simulink model "TrafficLights"  (R2023b)
settings: Solver=FixedStepAuto  StartTime=0.0  StopTime=50  FixedStep=1e-3  RelTol=1e-3  EnableMultiTasking=on
libraries: arduinolib x4
settings Model: ExtModeTrigDuration=2  Creator=MOHAMED  LastModifiedBy=MOHAMED
settings OptimizationCC: EnhancedBackFolding=on  PassReuseOutputArgsAs=Individual arguments  ZeroExternalMemoryAtStartup=off  ZeroInternalMemoryAtStartup=off  MaxStackSize=64  OptimizeBlockOrder=speed  DifferentSizesBufferReuse=on  OptimizationCustomize=off  EfficientTunableParamExpr=on
settings DebuggingCC: ParameterTunabilityLossMsg=error
settings HardwareCC: ProdBitPerInt=16  ProdBitPerPointer=16  ProdBitPerSizeT=16  ProdBitPerPtrDiffT=16  ProdLargestAtomicFloat=None  ProdWordSize=8  ProdHWDeviceType=Atmel->AVR
settings SFSimCC: MATLABDynamicMemAlloc=off
settings RTWCC: Description=Embedded Coder  SystemTargetFile=ert.tlc  HardwareBoard=Arduino Uno  TemplateMakefile=ert_default_tmf  Toolchain=Arduino AVR  BuildConfiguration=Faster Runs
settings CodeAppCC: ForceParamTrailComments=on  IgnoreCustomStorageClasses=off  OperatorAnnotations=on  SimulinkDataObjDesc=on  SFDataObjDesc=on  InsertBlockDesc=on
settings ERTTargetCC: SupportContinuousTime=on  SupportVariableSizeSignals=on  ExtModeTransport=3  ExtModeStaticAlloc=on  ExtModeAutomaticAllocSize=off  ExtModeStaticAllocSize=250  ExtModeMexFile=ext_xcp  ExtModeIntrfLevel=Level2 - Open

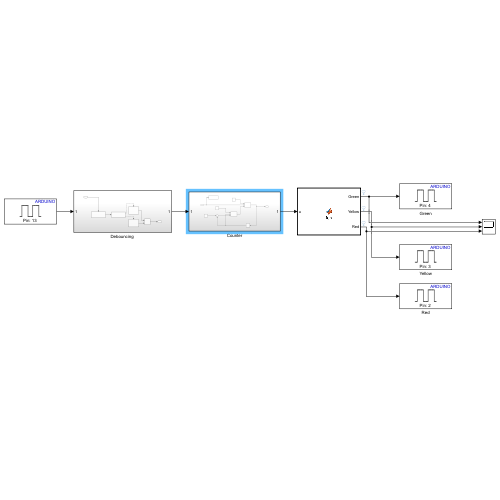
[thumbnail: Simulink's stored preview of the top-level diagram]
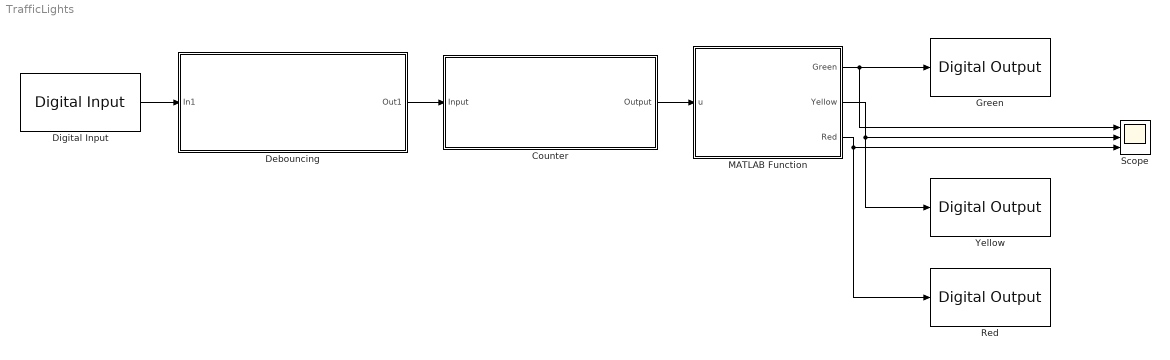
== system TrafficLights ==
  Counter : Subsystem
  "Debouncing " : Subsystem
  Digital Input : arduinolib/Digital Input  pinNumber=13  mode=Default  Direction=input  SampleTime=0.1  blockPlatform=arduino
  Green : arduinolib/Digital Output  pinNumber=4  Direction=output  blockPlatform=arduino
  MATLAB Function : MATLAB Function  TreatAsAtomicUnit=on
  Red : arduinolib/Digital Output  pinNumber=2  Direction=output  blockPlatform=arduino
  Scope : Scope  NumInputPorts=3
  Yellow : arduinolib/Digital Output  pinNumber=3  Direction=output  blockPlatform=arduino
  wires:
  Digital Input/1 -> "Debouncing "/1(In1)
  MATLAB Function/1(Green) -> Scope/1, Green/1
  "Debouncing "/1(Out1) -> Counter/1(Input)
  Counter/1(Output) -> MATLAB Function/1(u)
  MATLAB Function/3(Red) -> Red/1, Scope/3
  MATLAB Function/2(Yellow) -> Yellow/1, Scope/2

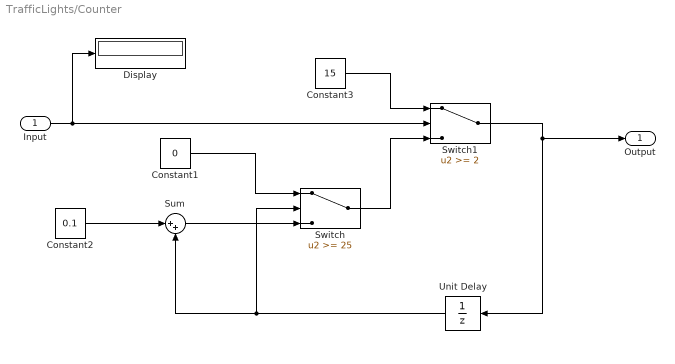
== system TrafficLights/Counter ==
  Input : Inport
  Constant1 : Constant  Value=0
  Constant2 : Constant  Value=0.1
  Constant3 : Constant  Value=15
  Display : Display
  Sum : Sum  Inputs=|++
  Switch : Switch  Threshold=25  SaturateOnIntegerOverflow=off  InputSameDT=off
  Switch1 : Switch  Threshold=2  SaturateOnIntegerOverflow=off  InputSameDT=off
  Unit Delay : UnitDelay  SampleTime=-1  HasFrameUpgradeWarning=on
  Output : Outport
  wires:
  Constant1/1 -> Switch/1
  Switch/1 -> Switch1/3
  Unit Delay/1 -> Switch/2, Sum/2
  Sum/1 -> Switch/3
  Constant2/1 -> Sum/1
  Switch1/1 -> Unit Delay/1, Output/1
  Input/1 -> Switch1/2, Display/1
  Constant3/1 -> Switch1/1

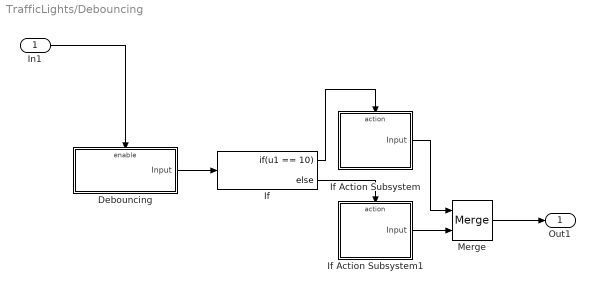
== system TrafficLights/Debouncing  ==
  In1 : Inport
  Debouncing : Subsystem  TreatAsAtomicUnit=on
  If : If  IfExpression=u1 == 10
  If Action Subsystem : Subsystem  TreatAsAtomicUnit=on
  If Action Subsystem1 : Subsystem  TreatAsAtomicUnit=on
  Merge : Merge
  Out1 : Outport
  wires:
  If Action Subsystem/1(Input) -> Merge/1
  Debouncing/1(Input) -> If/1
  Merge/1 -> Out1/1
  If Action Subsystem1/1(Input) -> Merge/2
  If/2 -> If Action Subsystem1/Action
  If/1 -> If Action Subsystem/Action
  In1/1 -> Debouncing/Enable

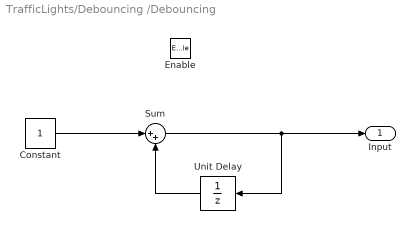
== system TrafficLights/Debouncing /Debouncing ==
  Enable : EnablePort  StatesWhenEnabling=reset
  Constant : Constant
  Sum : Sum  Inputs=|++
  Unit Delay : UnitDelay  SampleTime=-1  HasFrameUpgradeWarning=on
  Input : Outport
  wires:
  Sum/1 -> Unit Delay/1, Input/1
  Constant/1 -> Sum/1
  Unit Delay/1 -> Sum/2

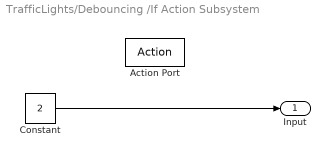
== system TrafficLights/Debouncing /If Action Subsystem ==
  Action Port : ActionPort  ActionPortLabel=if(u1 == 10)
  Constant : Constant  Value=2
  Input : Outport
  wires:
  Constant/1 -> Input/1

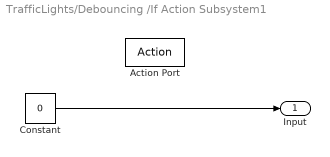
== system TrafficLights/Debouncing /If Action Subsystem1 ==
  Action Port : ActionPort  ActionPortLabel=else
  Constant : Constant  Value=0
  Input : Outport
  wires:
  Constant/1 -> Input/1

== matlab function TrafficLights/MATLAB Function ==
  data: u input; Green output; Yellow output; Red output
function [Green, Yellow, Red] = fcn(u)

Green = 0;
Yellow = 0;
Red = 0;

if (u >= 0 && u < 10)
    Green = 1;
    Yellow = 0;
    Red = 0;
elseif (u >= 10 && u < 15)
    Yellow = 1;
    Green = 0;
    Red = 0;
elseif (u >= 15 && u <= 25)
    Green = 0;
    Yellow = 0;
    Red = 1;
end
